simulink library "mfcm_block_lib_v1"  (Simulink 6.1)
undefined symbols (not defined in the file or in its folder): calc_path_data, mfcm_add_phase_noise, mfcm_delay_line_depth, mfcm_dpram_format_init, mfcm_dpram_format_lsb, mfcm_dpram_format_width, mfcm_matrix_rom, mfcm_phase_noise_pacc, mfcm_phase_noise_pinc, mfcm_spectrum_roms
libraries: xbsIndex_r4 x234, mfcm_misc_lib_v1 x8, mfcm_block_lib_v1 x4, mfcm_vector_lib_v1 x3, xbsCopyrightNotice_r4 x1
(part 3 of 3)

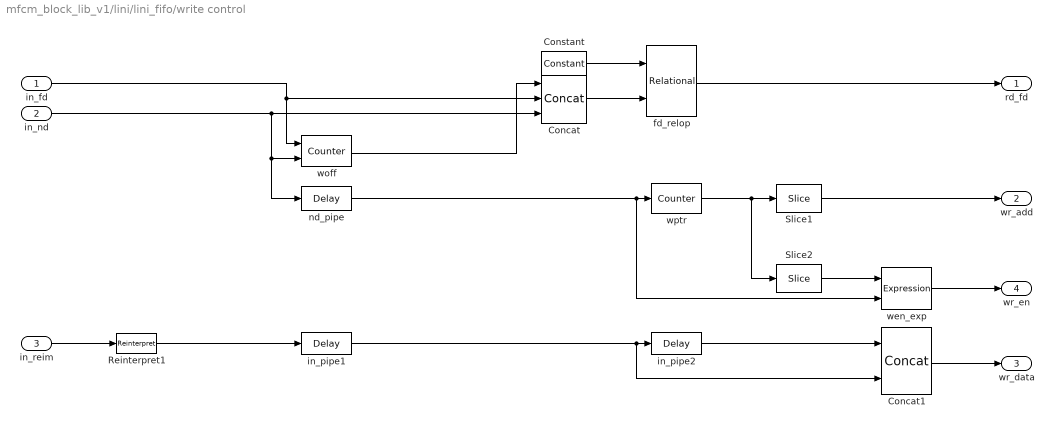
== system mfcm_block_lib_v1/lini/lini_fifo/write control ==
  in_fd : Inport  Port=1  LatchInput=off
  in_nd : Inport  Port=2  LatchInput=off
  in_reim : Inport  Port=3  LatchInput=off
  Concat : xbsIndex_r4/Concat  num_inputs=3  dbl_ovrd=off  block_type=concat
      settings: block_version=VER_STRING_GOES_HERE
  Concat1 : xbsIndex_r4/Concat  num_inputs=2  dbl_ovrd=off  block_type=concat
      settings: block_version=VER_STRING_GOES_HERE
  Constant : xbsIndex_r4/Constant  arith_type=Unsigned  const=4*(2*CHANNELS-2)+1  n_bits=ceil(log2(2*CHANNELS))+2  bin_pt=0  explicit_period=off  period=1  equ=P=C  opselect=C  inp2=PCIN>>17  opr=+  inp1=P  carry=CIN  dbl_ovrd=off  block_type=constant
      settings: block_version=VER_STRING_GOES_HERE
  Reinterpret1 : xbsIndex_r4/Reinterpret  force_arith_type=on  arith_type=Unsigned  force_bin_pt=on  bin_pt=0  block_type=cast
      settings: infoedit="Changes type of samples without altering their binary representation.<P><P>Hardware notes: In hardware this block costs nothing.<P><P>Example:  Suppose the input is 6 bits wide, signed, with 2 fractional bits, and the output is forced to unsigned with 0 fractional bits.  Then an input of -2.0 (1110.00 in binary 2's complement) becomes an output of 56 (111000 in binary)."  block_version=VER_STRING_GOES_HERE
  Slice1 : xbsIndex_r4/Slice  nbits=ceil(log2(4*CHANNELS))  boolean_output=off  mode=Upper Bit Location + Width  bit1=0  base1=MSB of Input  bit0=0  base0=LSB of Input  dbl_ovrd=off  block_type=slice
      settings: infoedit="Extracts a given range of bits from each input sample and presents it at the output.  The output type is ordinarily unsigned with binary point at zero, but can be Boolean when the slice is one bit wide.<P><P>Hardware notes: In hardware this block costs nothing."  block_version=VER_STRING_GOES_HERE
  Slice2 : xbsIndex_r4/Slice  nbits=1  boolean_output=on  mode=Lower Bit Location + Width  bit1=0  base1=MSB of Input  bit0=0  base0=LSB of Input  dbl_ovrd=off  block_type=slice
      settings: infoedit="Extracts a given range of bits from each input sample and presents it at the output.  The output type is ordinarily unsigned with binary point at zero, but can be Boolean when the slice is one bit wide.<P><P>Hardware notes: In hardware this block costs nothing."  block_version=VER_STRING_GOES_HERE
  fd_relop : xbsIndex_r4/Relational  mode=a=b  en=off  latency=1  dbl_ovrd=off  block_type=relational
      settings: xl_area=[0, 0, 0, 0, 0, 0, 0]  block_version=VER_STRING_GOES_HERE
  in_pipe1 : xbsIndex_r4/Delay  en=off  latency=1  dbl_ovrd=off  reg_retiming=off  block_type=delay
      settings: infoedit="Delay line having  configurable length.<P><P>Hardware notes: A delay line is a chain, each link of which is an SRL16 followed by a flip-flop. If register retiming is enabled, the delay line is a chain of flip-flops."  xl_area=[0, 0, 0, 0, 0, 0, 0]  block_version=VER_STRING_GOES_HERE
  in_pipe2 : xbsIndex_r4/Delay  en=off  latency=1  dbl_ovrd=off  reg_retiming=off  block_type=delay
      settings: infoedit="Delay line having  configurable length.<P><P>Hardware notes: A delay line is a chain, each link of which is an SRL16 followed by a flip-flop. If register retiming is enabled, the delay line is a chain of flip-flops."  xl_area=[0, 0, 0, 0, 0, 0, 0]  block_version=VER_STRING_GOES_HERE
  nd_pipe : xbsIndex_r4/Delay  en=off  latency=1  dbl_ovrd=off  reg_retiming=off  block_type=delay
      settings: infoedit="Delay line having  configurable length.<P><P>Hardware notes: A delay line is a chain, each link of which is an SRL16 followed by a flip-flop. If register retiming is enabled, the delay line is a chain of flip-flops."  xl_area=[0, 0, 0, 0, 0, 0, 0]  block_version=VER_STRING_GOES_HERE
  wen_exp : xbsIndex_r4/Expression  expression=~a & b  align_bp=on  en=off  latency=1  precision=Full  arith_type=Unsigned  n_bits=8  bin_pt=2  dbl_ovrd=off  block_type=expr
      settings: block_version=VER_STRING_GOES_HERE
  woff : xbsIndex_r4/Counter  cnt_type=Free Running  cnt_to=Inf  operation=Up  start_count=0  cnt_by_val=1  arith_type=Unsigned  n_bits=ceil(log2(2*CHANNELS))  bin_pt=0  load_pin=off  rst=on  en=on  dbl_ovrd=off  explicit_period=off  period=1  block_type=counter
      settings: infoedit="Configurable up, down and up/down counter.<P><P>Hardware notes: Free running counters are the least expensive in hardware.  A count limited counter is implemented by combining a counter with a comparator."  xl_area=[0, 0, 0, 0, 0, 0, 0]  block_version=VER_STRING_GOES_HERE
  wptr : xbsIndex_r4/Counter  cnt_type=Free Running  cnt_to=Inf  operation=Up  start_count=0  cnt_by_val=1  arith_type=Unsigned  n_bits=ceil(log2(4*CHANNELS))+1  bin_pt=0  load_pin=off  rst=off  en=on  dbl_ovrd=off  explicit_period=off  period=1  block_type=counter
      settings: infoedit="Configurable up, down and up/down counter.<P><P>Hardware notes: Free running counters are the least expensive in hardware.  A count limited counter is implemented by combining a counter with a comparator."  block_version=VER_STRING_GOES_HERE
  rd_fd : Outport
  wr_add : Outport  Port=2
  wr_data : Outport  Port=3
  wr_en : Outport  Port=4
  wires:
  woff/1 -> Concat/1
  Concat/1 -> fd_relop/2
  Constant/1 -> fd_relop/1
  fd_relop/1 -> rd_fd/1
  in_reim/1 -> Reinterpret1/1
  in_nd/1 -> woff/2, nd_pipe/1, Concat/3
  wptr/1 -> Slice1/1, Slice2/1
  in_fd/1 -> woff/1, Concat/2
  Slice1/1 -> wr_add/1
  in_pipe1/1 -> in_pipe2/1, Concat1/2
  Concat1/1 -> wr_data/1
  Reinterpret1/1 -> in_pipe1/1
  wen_exp/1 -> wr_en/1
  Slice2/1 -> wen_exp/1
  in_pipe2/1 -> Concat1/1
  nd_pipe/1 -> wptr/1, wen_exp/2

== system mfcm_block_lib_v1/phase_noise/pn_engine/counter ==
  rfd : Inport  Port=1  LatchInput=off
  Constant : xbsIndex_r4/Constant  arith_type=Signed (2's comp)  const=-2*N_OSC*prod(size(SPEC_DATA))  n_bits=1+ceil(log2(2*N_OSC*prod(size(SPEC_DATA))))  bin_pt=0  explicit_period=off  period=1  equ=P=C  opselect=C  inp2=PCIN>>17  opr=+  inp1=P  carry=CIN  dbl_ovrd=off  block_type=constant
      settings: block_version=VER_STRING_GOES_HERE
  Slice : xbsIndex_r4/Slice  nbits=ceil(log2(2*N_OSC*prod(size(SPEC_DATA))))  boolean_output=off  mode=Lower Bit Location + Width  bit1=0  base1=MSB of Input  bit0=0  base0=LSB of Input  dbl_ovrd=off  block_type=slice
      settings: infoedit="Extracts a given range of bits from each input sample and presents it at the output.  The output type is ordinarily unsigned with binary point at zero, but can be Boolean when the slice is one bit wide.<P><P>Hardware notes: In hardware this block costs nothing."  block_version=VER_STRING_GOES_HERE
  Slice1 : xbsIndex_r4/Slice  nbits=1  boolean_output=on  mode=Upper Bit Location + Width  bit1=0  base1=MSB of Input  bit0=0  base0=LSB of Input  dbl_ovrd=off  block_type=slice
      settings: infoedit="Extracts a given range of bits from each input sample and presents it at the output.  The output type is ordinarily unsigned with binary point at zero, but can be Boolean when the slice is one bit wide.<P><P>Hardware notes: In hardware this block costs nothing."  block_version=VER_STRING_GOES_HERE
  ce : xbsIndex_r4/Logical  logical_function=OR  inputs=2  en=off  latency=0  precision=Full  arith_type=Unsigned  n_bits=8  bin_pt=2  align_bp=on  dbl_ovrd=off  block_type=logical
      settings: block_version=VER_STRING_GOES_HERE
  count : xbsIndex_r4/Counter  cnt_type=Free Running  cnt_to=Inf  operation=Up  start_count=0  cnt_by_val=1  arith_type="Signed  (2's comp)"  n_bits=1+ceil(log2(2*N_OSC*prod(size(SPEC_DATA))))  bin_pt=0  load_pin=on  rst=off  en=on  dbl_ovrd=off  explicit_period=off  period=1  block_type=counter
      settings: infoedit="Configurable up, down and up/down counter.<P><P>Hardware notes: Free running counters are the least expensive in hardware.  A count limited counter is implemented by combining a counter with a comparator."  xl_area=[0, 0, 0, 0, 0, 0, 0]  block_version=VER_STRING_GOES_HERE
  run : Outport
  cnt : Outport  Port=2
  wires:
  count/1 -> Slice/1, Slice1/1
  Slice/1 -> cnt/1
  Slice1/1 -> run/1, ce/2
  rfd/1 -> count/1, ce/1
  Constant/1 -> count/2
  ce/1 -> count/3

== system mfcm_block_lib_v1/phase_noise/pn_engine/noise_rom ==
  note: If the ROM contains the same value, the mux translates
      | the ROM into a constant
  path : Inport  Port=1  LatchInput=off
  Constant : xbsIndex_r4/Constant  arith_type=Boolean  const=double(min([SPEC_DATA.noise])==max([SPEC_DATA.noise]))  n_bits=1  bin_pt=0  explicit_period=off  period=1  equ=P=C  opselect=C  inp2=PCIN>>17  opr=+  inp1=P  carry=CIN  dbl_ovrd=off  block_type=constant
      settings: block_version=VER_STRING_GOES_HERE
  Constant2 : xbsIndex_r4/Constant  arith_type=Boolean  const=double(max([SPEC_DATA.noise]))  n_bits=1  bin_pt=0  explicit_period=off  period=1  equ=P=C  opselect=C  inp2=PCIN>>17  opr=+  inp1=P  carry=CIN  dbl_ovrd=off  block_type=constant
      settings: block_version=VER_STRING_GOES_HERE
  Mux : xbsIndex_r4/Mux  inputs=2  en=off  latency=0  precision=Full  arith_type=Unsigned  n_bits=8  bin_pt=2  quantization=Truncate  overflow=Wrap  dbl_ovrd=off  block_type=mux
      settings: block_version=VER_STRING_GOES_HERE
  noise_rom : xbsIndex_r4/ROM  depth=2^ceil(log2(max(prod(size(SPEC_DATA)),2)))  initVector=double([SPEC_DATA.noise])  distributed_mem=Distributed memory  rst=off  init_reg=0  en=off  latency=1  arith_type=Boolean  n_bits=18  bin_pt=17  dbl_ovrd=off  use_rpm=off  block_type=sprom
      settings: xl_area=[0, 0, 0, 0, 0, 0, 0]  block_version=VER_STRING_GOES_HERE
  flag : Outport
  wires:
  Constant/1 -> Mux/1
  noise_rom/1 -> Mux/2
  Constant2/1 -> Mux/3
  Mux/1 -> flag/1
  path/1 -> noise_rom/1

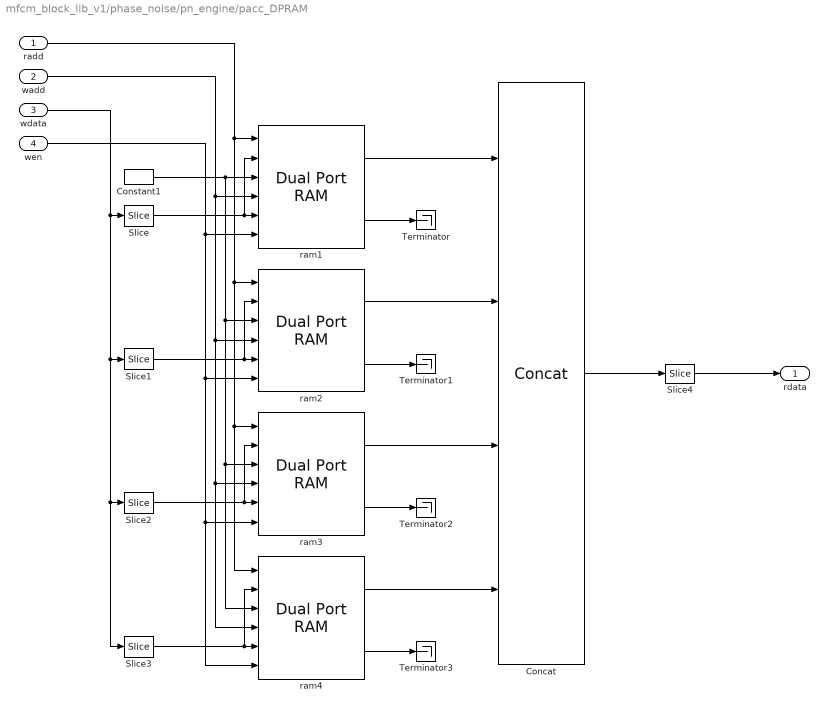
== system mfcm_block_lib_v1/phase_noise/pn_engine/pacc_DPRAM ==
  radd : Inport  Port=1  LatchInput=off
  wadd : Inport  Port=2  LatchInput=off
  wdata : Inport  Port=3  LatchInput=off
  wen : Inport  Port=4  LatchInput=off
  Concat : xbsIndex_r4/Concat  num_inputs=4  dbl_ovrd=off  block_type=concat
      settings: block_version=VER_STRING_GOES_HERE
  Constant1 : xbsIndex_r4/Constant  arith_type=Boolean  const=0  n_bits=1  bin_pt=0  explicit_period=off  period=1  equ=P=C  opselect=C  inp2=PCIN>>17  opr=+  inp1=P  carry=CIN  dbl_ovrd=off  block_type=constant
      settings: block_version=VER_STRING_GOES_HERE
  Slice : xbsIndex_r4/Slice  nbits=mfcm_dpram_format_width(1,4,MEM_DEPTH,OUT_WIDTH,MEM_INIT)  boolean_output=off  mode=Lower Bit Location + Width  bit1=0  base1=MSB of Input  bit0=mfcm_dpram_format_lsb(1,4,MEM_DEPTH,OUT_WIDTH,MEM_INIT)  base0=LSB of Input  dbl_ovrd=off  block_type=slice
      settings: infoedit="Extracts a given range of bits from each input sample and presents it at the output.  The output type is ordinarily unsigned with binary point at zero, but can be Boolean when the slice is one bit wide.<P><P>Hardware notes: In hardware this block costs nothing."  block_version=VER_STRING_GOES_HERE
  Slice1 : xbsIndex_r4/Slice  nbits=mfcm_dpram_format_width(2,4,MEM_DEPTH,OUT_WIDTH,MEM_INIT)  boolean_output=off  mode=Lower Bit Location + Width  bit1=0  base1=MSB of Input  bit0=mfcm_dpram_format_lsb(2,4,MEM_DEPTH,OUT_WIDTH,MEM_INIT)  base0=LSB of Input  dbl_ovrd=off  block_type=slice
      settings: infoedit="Extracts a given range of bits from each input sample and presents it at the output.  The output type is ordinarily unsigned with binary point at zero, but can be Boolean when the slice is one bit wide.<P><P>Hardware notes: In hardware this block costs nothing."  block_version=VER_STRING_GOES_HERE
  Slice2 : xbsIndex_r4/Slice  nbits=mfcm_dpram_format_width(3,4,MEM_DEPTH,OUT_WIDTH,MEM_INIT)  boolean_output=off  mode=Lower Bit Location + Width  bit1=0  base1=MSB of Input  bit0=mfcm_dpram_format_lsb(3,4,MEM_DEPTH,OUT_WIDTH,MEM_INIT)  base0=LSB of Input  dbl_ovrd=off  block_type=slice
      settings: infoedit="Extracts a given range of bits from each input sample and presents it at the output.  The output type is ordinarily unsigned with binary point at zero, but can be Boolean when the slice is one bit wide.<P><P>Hardware notes: In hardware this block costs nothing."  block_version=VER_STRING_GOES_HERE
  Slice3 : xbsIndex_r4/Slice  nbits=mfcm_dpram_format_width(4,4,MEM_DEPTH,OUT_WIDTH,MEM_INIT)  boolean_output=off  mode=Lower Bit Location + Width  bit1=0  base1=MSB of Input  bit0=mfcm_dpram_format_lsb(4,4,MEM_DEPTH,OUT_WIDTH,MEM_INIT)  base0=LSB of Input  dbl_ovrd=off  block_type=slice
      settings: infoedit="Extracts a given range of bits from each input sample and presents it at the output.  The output type is ordinarily unsigned with binary point at zero, but can be Boolean when the slice is one bit wide.<P><P>Hardware notes: In hardware this block costs nothing."  block_version=VER_STRING_GOES_HERE
  Slice4 : xbsIndex_r4/Slice  nbits=OUT_WIDTH  boolean_output=off  mode=Upper Bit Location + Width  bit1=0  base1=MSB of Input  bit0=0  base0=LSB of Input  dbl_ovrd=off  block_type=slice
      settings: infoedit="Extracts a given range of bits from each input sample and presents it at the output.  The output type is ordinarily unsigned with binary point at zero, but can be Boolean when the slice is one bit wide.<P><P>Hardware notes: In hardware this block costs nothing."  block_version=VER_STRING_GOES_HERE
  Terminator{,1..3} (4 alike) : Terminator
  ram1 : xbsIndex_r4/Dual Port RAM  depth=MEM_DEPTH  initVector=mfcm_dpram_format_init(1,4,MEM_DEPTH,OUT_WIDTH,MEM_INIT)  distributed_mem=Block RAM  init_a=0  init_b=0  rst_a=off  rst_b=off  en_a=off  en_b=off  latency=2  write_mode_A=Read After Write  write_mode_B=Read After Write  dbl_ovrd=off  use_rpm=on  block_type=dpram
      settings: block_version=VER_STRING_GOES_HERE
  ram2 : xbsIndex_r4/Dual Port RAM  depth=MEM_DEPTH  initVector=mfcm_dpram_format_init(2,4,MEM_DEPTH,OUT_WIDTH,MEM_INIT)  distributed_mem=Block RAM  init_a=0  init_b=0  rst_a=off  rst_b=off  en_a=off  en_b=off  latency=2  write_mode_A=Read After Write  write_mode_B=Read After Write  dbl_ovrd=off  use_rpm=on  block_type=dpram
      settings: block_version=VER_STRING_GOES_HERE
  ram3 : xbsIndex_r4/Dual Port RAM  depth=MEM_DEPTH  initVector=mfcm_dpram_format_init(3,4,MEM_DEPTH,OUT_WIDTH,MEM_INIT)  distributed_mem=Block RAM  init_a=0  init_b=0  rst_a=off  rst_b=off  en_a=off  en_b=off  latency=2  write_mode_A=Read After Write  write_mode_B=Read After Write  dbl_ovrd=off  use_rpm=on  block_type=dpram
      settings: block_version=VER_STRING_GOES_HERE
  ram4 : xbsIndex_r4/Dual Port RAM  depth=MEM_DEPTH  initVector=mfcm_dpram_format_init(4,4,MEM_DEPTH,OUT_WIDTH,MEM_INIT)  distributed_mem=Block RAM  init_a=0  init_b=0  rst_a=off  rst_b=off  en_a=off  en_b=off  latency=2  write_mode_A=Read After Write  write_mode_B=Read After Write  dbl_ovrd=off  use_rpm=on  block_type=dpram
      settings: block_version=VER_STRING_GOES_HERE
  rdata : Outport
  wires:
  Slice4/1 -> rdata/1
  Concat/1 -> Slice4/1
  ram4/1 -> Concat/4
  ram3/1 -> Concat/3
  ram2/1 -> Concat/2
  ram1/1 -> Concat/1
  ram3/2 -> Terminator2/1
  ram4/2 -> Terminator3/1
  ram2/2 -> Terminator1/1
  ram1/2 -> Terminator/1
  wen/1 -> ram3/6, ram4/6, ram2/6, ram1/6
  wdata/1 -> Slice/1, Slice1/1, Slice2/1, Slice3/1
  wadd/1 -> ram3/4, ram4/4, ram2/4, ram1/4
  radd/1 -> ram3/1, ram4/1, ram2/1, ram1/1
  Constant1/1 -> ram3/3, ram4/3, ram2/3, ram1/3
  Slice3/1 -> ram4/5, ram4/2
  Slice2/1 -> ram3/5, ram3/2
  Slice1/1 -> ram2/5, ram2/2
  Slice/1 -> ram1/5, ram1/2

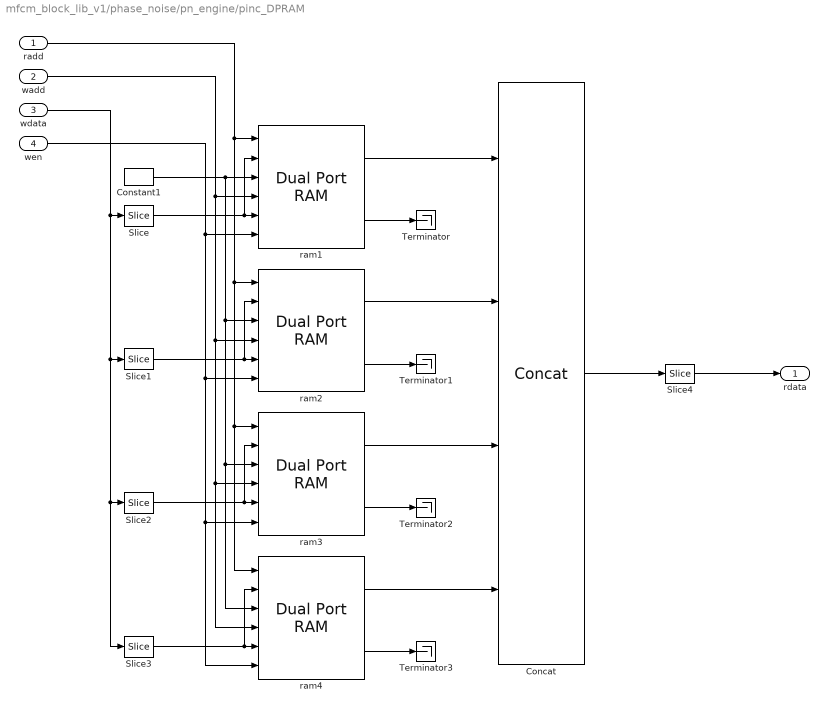
== system mfcm_block_lib_v1/phase_noise/pn_engine/pinc_DPRAM ==
  radd : Inport  Port=1  LatchInput=off
  wadd : Inport  Port=2  LatchInput=off
  wdata : Inport  Port=3  LatchInput=off
  wen : Inport  Port=4  LatchInput=off
  Concat : xbsIndex_r4/Concat  num_inputs=4  dbl_ovrd=off  block_type=concat
      settings: block_version=VER_STRING_GOES_HERE
  Constant1 : xbsIndex_r4/Constant  arith_type=Boolean  const=0  n_bits=1  bin_pt=0  explicit_period=off  period=1  equ=P=C  opselect=C  inp2=PCIN>>17  opr=+  inp1=P  carry=CIN  dbl_ovrd=off  block_type=constant
      settings: block_version=VER_STRING_GOES_HERE
  Slice : xbsIndex_r4/Slice  nbits=mfcm_dpram_format_width(1,4,MEM_DEPTH,OUT_WIDTH,MEM_INIT)  boolean_output=off  mode=Lower Bit Location + Width  bit1=0  base1=MSB of Input  bit0=mfcm_dpram_format_lsb(1,4,MEM_DEPTH,OUT_WIDTH,MEM_INIT)  base0=LSB of Input  dbl_ovrd=off  block_type=slice
      settings: infoedit="Extracts a given range of bits from each input sample and presents it at the output.  The output type is ordinarily unsigned with binary point at zero, but can be Boolean when the slice is one bit wide.<P><P>Hardware notes: In hardware this block costs nothing."  block_version=VER_STRING_GOES_HERE
  Slice1 : xbsIndex_r4/Slice  nbits=mfcm_dpram_format_width(2,4,MEM_DEPTH,OUT_WIDTH,MEM_INIT)  boolean_output=off  mode=Lower Bit Location + Width  bit1=0  base1=MSB of Input  bit0=mfcm_dpram_format_lsb(2,4,MEM_DEPTH,OUT_WIDTH,MEM_INIT)  base0=LSB of Input  dbl_ovrd=off  block_type=slice
      settings: infoedit="Extracts a given range of bits from each input sample and presents it at the output.  The output type is ordinarily unsigned with binary point at zero, but can be Boolean when the slice is one bit wide.<P><P>Hardware notes: In hardware this block costs nothing."  block_version=VER_STRING_GOES_HERE
  Slice2 : xbsIndex_r4/Slice  nbits=mfcm_dpram_format_width(3,4,MEM_DEPTH,OUT_WIDTH,MEM_INIT)  boolean_output=off  mode=Lower Bit Location + Width  bit1=0  base1=MSB of Input  bit0=mfcm_dpram_format_lsb(3,4,MEM_DEPTH,OUT_WIDTH,MEM_INIT)  base0=LSB of Input  dbl_ovrd=off  block_type=slice
      settings: infoedit="Extracts a given range of bits from each input sample and presents it at the output.  The output type is ordinarily unsigned with binary point at zero, but can be Boolean when the slice is one bit wide.<P><P>Hardware notes: In hardware this block costs nothing."  block_version=VER_STRING_GOES_HERE
  Slice3 : xbsIndex_r4/Slice  nbits=mfcm_dpram_format_width(4,4,MEM_DEPTH,OUT_WIDTH,MEM_INIT)  boolean_output=off  mode=Lower Bit Location + Width  bit1=0  base1=MSB of Input  bit0=mfcm_dpram_format_lsb(4,4,MEM_DEPTH,OUT_WIDTH,MEM_INIT)  base0=LSB of Input  dbl_ovrd=off  block_type=slice
      settings: infoedit="Extracts a given range of bits from each input sample and presents it at the output.  The output type is ordinarily unsigned with binary point at zero, but can be Boolean when the slice is one bit wide.<P><P>Hardware notes: In hardware this block costs nothing."  block_version=VER_STRING_GOES_HERE
  Slice4 : xbsIndex_r4/Slice  nbits=OUT_WIDTH  boolean_output=off  mode=Upper Bit Location + Width  bit1=0  base1=MSB of Input  bit0=0  base0=LSB of Input  dbl_ovrd=off  block_type=slice
      settings: infoedit="Extracts a given range of bits from each input sample and presents it at the output.  The output type is ordinarily unsigned with binary point at zero, but can be Boolean when the slice is one bit wide.<P><P>Hardware notes: In hardware this block costs nothing."  block_version=VER_STRING_GOES_HERE
  Terminator{,1..3} (4 alike) : Terminator
  ram1 : xbsIndex_r4/Dual Port RAM  depth=MEM_DEPTH  initVector=mfcm_dpram_format_init(1,4,MEM_DEPTH,OUT_WIDTH,MEM_INIT)  distributed_mem=Block RAM  init_a=0  init_b=0  rst_a=off  rst_b=off  en_a=off  en_b=off  latency=2  write_mode_A=Read After Write  write_mode_B=Read After Write  dbl_ovrd=off  use_rpm=on  block_type=dpram
      settings: block_version=VER_STRING_GOES_HERE
  ram2 : xbsIndex_r4/Dual Port RAM  depth=MEM_DEPTH  initVector=mfcm_dpram_format_init(2,4,MEM_DEPTH,OUT_WIDTH,MEM_INIT)  distributed_mem=Block RAM  init_a=0  init_b=0  rst_a=off  rst_b=off  en_a=off  en_b=off  latency=2  write_mode_A=Read After Write  write_mode_B=Read After Write  dbl_ovrd=off  use_rpm=on  block_type=dpram
      settings: block_version=VER_STRING_GOES_HERE
  ram3 : xbsIndex_r4/Dual Port RAM  depth=MEM_DEPTH  initVector=mfcm_dpram_format_init(3,4,MEM_DEPTH,OUT_WIDTH,MEM_INIT)  distributed_mem=Block RAM  init_a=0  init_b=0  rst_a=off  rst_b=off  en_a=off  en_b=off  latency=2  write_mode_A=Read After Write  write_mode_B=Read After Write  dbl_ovrd=off  use_rpm=on  block_type=dpram
      settings: block_version=VER_STRING_GOES_HERE
  ram4 : xbsIndex_r4/Dual Port RAM  depth=MEM_DEPTH  initVector=mfcm_dpram_format_init(4,4,MEM_DEPTH,OUT_WIDTH,MEM_INIT)  distributed_mem=Block RAM  init_a=0  init_b=0  rst_a=off  rst_b=off  en_a=off  en_b=off  latency=2  write_mode_A=Read After Write  write_mode_B=Read After Write  dbl_ovrd=off  use_rpm=on  block_type=dpram
      settings: block_version=VER_STRING_GOES_HERE
  rdata : Outport
  wires:
  Slice/1 -> ram1/5, ram1/2
  Slice1/1 -> ram2/5, ram2/2
  Slice2/1 -> ram3/5, ram3/2
  Slice3/1 -> ram4/5, ram4/2
  Constant1/1 -> ram3/3, ram4/3, ram2/3, ram1/3
  radd/1 -> ram3/1, ram4/1, ram2/1, ram1/1
  wadd/1 -> ram3/4, ram4/4, ram2/4, ram1/4
  wdata/1 -> Slice3/1, Slice2/1, Slice1/1, Slice/1
  wen/1 -> ram3/6, ram4/6, ram2/6, ram1/6
  ram1/2 -> Terminator/1
  ram2/2 -> Terminator1/1
  ram4/2 -> Terminator3/1
  ram3/2 -> Terminator2/1
  ram1/1 -> Concat/1
  ram2/1 -> Concat/2
  ram3/1 -> Concat/3
  ram4/1 -> Concat/4
  Concat/1 -> Slice4/1
  Slice4/1 -> rdata/1

== system mfcm_block_lib_v1/phase_noise/pn_engine/pn_acc ==
  note: Wide accumulator taking 2 cycles.
      | LSBs presented first, then MSBs with carry from first add
  note: The natural way to do this is as an a+b+cin add block,
      | but this should hopefully absorbe all the mux logic into the adder LUTs
      | The fudge blocks propogate sample times
  msb_not_lsb : Inport  Port=1  LatchInput=off
  inc_in : Inport  Port=2  LatchInput=off
  acc_in : Inport  Port=3  LatchInput=off
  Convert : xbsIndex_r4/Convert  arith_type=Unsigned  n_bits=1  bin_pt=0  quantization=Truncate  overflow=Wrap  latency=0  dbl_ovrd=off  pipeline=off  block_type=convert
      settings: infoedit=The input is presented at the output after quantization and overflow effects.<P><P>Hardware notes: Additional hardware is used when rounding or saturation is selected and output width is less than the input width.  xl_area=[0, 0, 0, 0, 0, 0, 0]  block_version=VER_STRING_GOES_HERE
  Mux : xbsIndex_r4/Mux  inputs=2  en=off  latency=0  precision=Full  arith_type=Unsigned  n_bits=8  bin_pt=2  quantization=Truncate  overflow=Wrap  dbl_ovrd=off  block_type=mux
      settings: block_version=VER_STRING_GOES_HERE
  acc : xbsIndex_r4/AddSub  mode=Addition  use_carryin=off  use_carryout=on  en=off  latency=1  precision=User Defined  arith_type=Unsigned  n_bits=log2(N_IDFT)  bin_pt=0  quantization=Truncate  overflow=Wrap  dbl_ovrd=off  use_behavioral_HDL=on  pipelined=off  use_rpm=off  block_type=addsub
      settings: xl_area=[0, 0, 0, 0, 0, 0, 0]  block_version=VER_STRING_GOES_HERE
  fudge : xbsIndex_r4/Logical  logical_function=OR  inputs=2  en=off  latency=0  precision=Full  arith_type=Unsigned  n_bits=8  bin_pt=2  align_bp=on  dbl_ovrd=off  block_type=logical
      settings: xl_area=[0, 0, 0, 0, 0, 0, 0]  block_version=VER_STRING_GOES_HERE
  fudge1 : xbsIndex_r4/Logical  logical_function=XOR  inputs=2  en=off  latency=0  precision=Full  arith_type=Unsigned  n_bits=8  bin_pt=2  align_bp=on  dbl_ovrd=off  block_type=logical
      settings: xl_area=[0, 0, 0, 0, 0, 0, 0]  block_version=VER_STRING_GOES_HERE
  acc_out : Outport
  wires:
  acc_in/1 -> acc/1
  acc/1 -> acc_out/1
  msb_not_lsb/1 -> Convert/1, Mux/1
  inc_in/1 -> Mux/2
  Mux/1 -> acc/2
  Convert/1 -> fudge1/1, fudge1/2
  fudge/1 -> Mux/3
  fudge1/1 -> fudge/1  "always 0"
  acc/2 -> fudge/2

== system mfcm_block_lib_v1/lini/lini_fifo/read control/wait for valid ==
  note: We need at least two valid blocks in the FIFO before we can interpolate.
      | This shift register checks this condition
  rd_fd : Inport  Port=1  LatchInput=off
  pn_rfd : Inport  Port=2  LatchInput=off
  Register : xbsIndex_r4/Register  init=0  rst=off  en=on  dbl_ovrd=off  block_type=register
      settings: xl_area=[0, 0, 0, 0, 0, 0, 0]  block_version=VER_STRING_GOES_HERE
  Register1 : xbsIndex_r4/Register  init=0  rst=off  en=on  dbl_ovrd=off  block_type=register
      settings: xl_area=[0, 0, 0, 0, 0, 0, 0]  block_version=VER_STRING_GOES_HERE
  Register2 : xbsIndex_r4/Register  init=0  rst=off  en=on  dbl_ovrd=off  block_type=register
      settings: xl_area=[0, 0, 0, 0, 0, 0, 0]  block_version=VER_STRING_GOES_HERE
  valid : Outport
  wires:
  Register1/1 -> valid/1
  rd_fd/1 -> Register2/2, Register/2, Register/1
  pn_rfd/1 -> Register1/2
  Register/1 -> Register2/1
  Register2/1 -> Register1/1
